simulink model "UAV_model_control"  (R2023a)
settings: Solver=VariableStepAuto  StartTime=0.0  StopTime=10.0  RelTol=1e-3
values from neighbouring files (symbols this model uses):
  b = 0.001    [model_params.m]
  Dt = [1 0 -sin(th(2)) ... (first row only)    [model_params.m]
  Fb = k * [0; 0; sum(rho.^2)]    [model_params.m]
  Fd = -D * [p_dot(1); p_dot(2); p_dot(3)]    [model_params.m]
  g = 9.80665    [environment_variables.m]    (also in model_params.m = [0; 0; -9.81]; uas_parameters.m)
  I = diag([Ixx, Iyy, Izz])    [model_params.m]
  Ixx = 3*10^-6    (= 3e-06)    [model_params.m]
  Iyy = Ixx    (= 3e-06)    [model_params.m]
  Izz = 1*10^-5    (= 1e-05)    [model_params.m]
  k = 0.01    [model_params.m]
  L = 0.225    [model_params.m]
  m = 0.5    [model_params.m]
  R = Rz * Ry * Rx    [model_params.m]
undefined symbols (not defined in the file or in its folder): Theta
libraries: aerolibutil x2, Contact_Forces_Lib x1, slpidlib x1
settings Model: Creator=dcest  LastModifiedBy=jonas
settings OptimizationCC: ReuseModelBlockBuffer=off

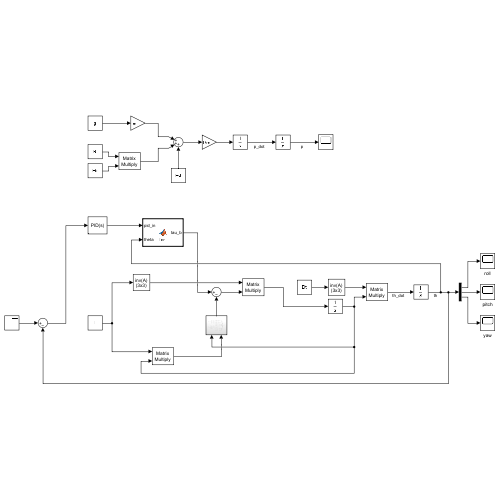
[thumbnail: Simulink's stored preview of the top-level diagram]
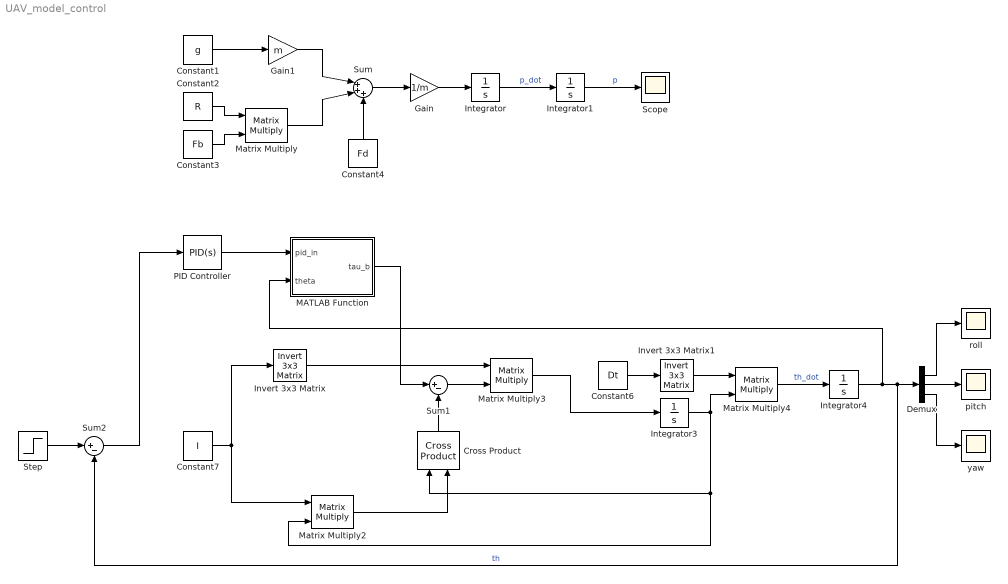
== system UAV_model_control ==
  Constant1 : Constant  Value=g
  Constant2 : Constant  Value=R
  Constant3 : Constant  Value=Fb
  Constant4 : Constant  Value=Fd
  Constant6 : Constant  Value=Dt
  Constant7 : Constant  Value=I
  Cross Product : Contact_Forces_Lib/Math/Cross Product  SystemSampleTime=-1  VariantActivationTime=update diagram  Latency=0  AutoFrameSizeCalculation=off
      settings: SourceProductName=Simscape Multibody Contact Forces Library
  Demux : Demux  Outputs=3
  Gain : Gain  Gain=1/m
  Gain1 : Gain  Gain=m
  Integrator{,1,3..4} (4 alike) : Integrator
  Invert 3x3 Matrix : aerolibutil/Invert  3x3 Matrix
  Invert 3x3 Matrix1 : aerolibutil/Invert  3x3 Matrix
  MATLAB Function : MATLAB Function  TreatAsAtomicUnit=on
  Matrix Multiply{,2..4} (4 alike) : Product  Multiplication=Matrix(*)
  PID Controller : slpidlib/PID Controller  Controller=PID  Form=Parallel  TimeDomain=Continuous-time  UseExternalTs=off  SampleTime=-1  IntegratorMethod=Forward Euler  FilterMethod=Forward Euler  ControllerParametersSource=internal  P=1  I=0  UseKiTs=off  D=0  N=100  UseFilter=on  TunerSelectOption=Transfer Function Based (PID Tuner App)  InitialConditionSource=internal  InitialConditionForIntegrator=0  InitialConditionForFilter=0  DifferentiatorICPrevScaledInput=0  ExternalReset=none  TrackingMode=off  Kt=1  LimitOutput=off  SatLimitsSource=internal  UpperSaturationLimit=inf  LowerSaturationLimit=-inf  LinearizeAsGain=on  AntiWindupMode=none  Kb=1  LimitIntegrator=off  UpperIntegratorSaturationLimit=inf  LowerIntegratorSaturationLimit=-inf  POutMin=[]  POutMax=[]  IOutMin=[]  IOutMax=[]  DOutMin=[]  DOutMax=[]  NOutMin=[]  NOutMax=[]  SumOutMin=[]  SumOutMax=[]  SaturationOutMin=[]  SaturationOutMax=[]  PParamMin=[]  PParamMax=[]  IParamMin=[]  IParamMax=[]  DParamMin=[]  DParamMax=[]  NParamMin=[]  NParamMax=[]  KbParamMin=[]  KbParamMax=[]  KtParamMin=[]  KtParamMax=[]  KbOutMin=[]  KbOutMax=[]  KtOutMin=[]  KtOutMax=[]  IntegratorOutMin=[]  IntegratorOutMax=[]  FilterOutMin=[]  FilterOutMax=[]  SumI1OutMin=[]  SumI1OutMax=[]  SumI2OutMin=[]  SumI2OutMax=[]  SumI3OutMin=[]  SumI3OutMax=[]  SumI4OutMin=[]  SumI4OutMax=[]  SumDOutMin=[]  SumDOutMax=[]  DifferentiatorOutMin=[]  DifferentiatorOutMax=[]  FilterDiffOutCoefMin=[]  FilterDiffOutCoefMax=[]  ReciprocalOutMin=[]  ReciprocalOutMax=[]  SumDenOutMin=[]  SumDenOutMax=[]  SumNumOutMin=[]  SumNumOutMax=[]  DivideOutMin=[]  DivideOutMax=[]  UdiffTsProdOutMin=[]  UdiffTsProdOutMax=[]  NTsProdOutMin=[]  NTsProdOutMax=[]  UintegralTsProdOutMin=[]  UintegralTsProdOutMax=[]  UngainTsProdOutMin=[]  UngainTsProdOutMax=[]  ClampingZeroOutDataTypeStr=Inherit: Inherit via back propagation  ClampingZeroOutMin=[]  ClampingZeroOutMax=[]  FilterDenConstantOutDataTypeStr=Inherit: Inherit via back propagation  FilterDenConstantOutMin=[]  FilterDenConstantOutMax=[]  PCopyOutDataTypeStr=Inherit: Inherit via back propagation  PCopyOutMin=[]  PCopyOutMax=[]  NCopyOutDataTypeStr=Inherit: Inherit via back propagation  NCopyOutMin=[]  NCopyOutMax=[]  IntegratorContinuousStateAttributes=''  IntegratorStateMustResolveToSignalObject=off  IntegratorRTWStateStorageClass=Auto  FilterContinuousStateAttributes=''  FilterStateMustResolveToSignalObject=off  FilterRTWStateStorageClass=Auto  ParallelPVariant=InternalParameters  IdealPVariant=Disabled  IVariant=InternalParameters  DVariant=InternalParameters  IntegratorVariant=Continuous  SatVariant=Disabled  AWVariant=Passthrough  PCopyVariant=Disabled  TRVariant=Disabled  FdbkBlocksVariant=Forward  IdealPFdbkVariant=Disabled  SatFdbkVariant=Disabled  DerivativeFilterVariant=ContFilter  NVariant=InternalParameters  NCopyVariant=Disabled  FilterICVariant=InternalICsFilter  IntegratorICVariant=InternalICs  ExternalResetVariant=Disabled  TRSumVariant=Passthrough  SumFdbkVariant=Disabled  SumVariant=Sum_PID  TsampFilterVariant=InternalTs  TsampNgainVariant=Passthrough  TsampIntegralVariant=Disabled_SignalSpec  ExternalSaturationOutDataTypeStr=Inherit: Same as second input
  Scope : Scope
  Step : Step  After=Theta  SampleTime=0  VectorParams1D=off
  Sum : Sum  Inputs=|+++
  Sum1 : Sum  Inputs=|+-
  Sum2 : Sum  Inputs=|+-
  pitch : Scope
  roll : Scope
  yaw : Scope
  wires:
  Constant2/1 -> Matrix Multiply/1
  Constant3/1 -> Matrix Multiply/2
  Matrix Multiply/1 -> Sum/2
  Constant4/1 -> Sum/3
  Sum/1 -> Gain/1
  Gain/1 -> Integrator/1
  Constant7/1 -> Matrix Multiply2/1, Invert 3x3 Matrix/1
  Matrix Multiply2/1 -> Cross Product/2
  MATLAB Function/1(tau_b) -> Sum1/1
  Cross Product/1 -> Sum1/2
  Invert 3x3 Matrix/1 -> Matrix Multiply3/1
  Sum1/1 -> Matrix Multiply3/2
  Matrix Multiply3/1 -> Integrator3/1
  Integrator3/1 -> Matrix Multiply2/2, Cross Product/1, Matrix Multiply4/2
  Constant6/1 -> Invert 3x3 Matrix1/1
  Invert 3x3 Matrix1/1 -> Matrix Multiply4/1
  Constant1/1 -> Gain1/1
  Gain1/1 -> Sum/1
  Integrator1/1 -> Scope/1  "p"
  Integrator/1 -> Integrator1/1  "p_dot"
  Matrix Multiply4/1 -> Integrator4/1  "th_dot"
  Integrator4/1 -> MATLAB Function/2(theta), Sum2/2, Demux/1  "th"
  Step/1 -> Sum2/1
  Sum2/1 -> PID Controller/1
  PID Controller/1 -> MATLAB Function/1(pid_in)
  Demux/2 -> pitch/1
  Demux/3 -> yaw/1
  Demux/1 -> roll/1

== matlab function UAV_model_control/MATLAB Function ==
  data: pid_in input; theta input; tau_b output; k parameter; m parameter; g parameter; b parameter; Ixx parameter; Iyy parameter; Izz parameter; L parameter
function tau_b = fcn(pid_in, theta, k, m, g, b, Ixx, Iyy, Izz, L)
    theta = theta + [0;0;0];

    u_phi = pid_in(1);
    u_theta = pid_in(2);
    u_psi = pid_in(3);

    add_0 = (m*g(3))/(k*4*cos(theta(2))*cos(theta(1)));

    add_1 = -(2*b*u_phi*Ixx+u_psi*Izz*k*L)/(4*b*k*L);
    add_2 = -(2*b*u_theta*Iyy-u_psi*Izz*k*L)/(4*b*k*L);
    add_3 = -(-2*b*u_phi*Ixx+u_psi*Izz*k*L)/(4*b*k*L);
    add_4 = -(-2*b*u_theta*Iyy-u_psi*Izz*k*L)/(4*b*k*L);

    gamma_1 = add_0 + add_1;
    gamma_2 = add_0 + add_2;
    gamma_3 = add_0 + add_3;
    gamma_4 = add_0 + add_4;

    tau_b = [L*k*(gamma_1-gamma_3) ; L*k*(gamma_2-gamma_4) ; b*(gamma_1-gamma_2+gamma_3-gamma_4)];
